simulink library "asbhl20act"  (R2016b)
settings: Solver=ode45  StartTime=0.0  StopTime=10.0  RelTol=1e-3
undefined symbols (not defined in the file): max_lim, min_lim
libraries: aerolibactuator x13, simulink x12
Description:
  | HL-20 control surface actuators component module
  | 
  | Copyright 1990-2007 The MathWorks Inc.
settings Model: Creator=The MathWorks, Inc.  LastModifiedBy=The MathWorks, Inc.
settings DataIOCC: LimitDataPoints=on  SaveFormat=Array  SignalLoggingSaveFormat=ModelDataLogs
settings OptimizationCC: BlockReduction=off  BooleanDataType=off  ExpressionDepthLimit=2147483647  LifeSpan=inf
settings DebuggingCC: SaveWithParameterizedLinksMsg=none  UnderspecifiedInitializationDetection=Classic  MergeDetectMultiDrivingBlocksExec=none  SignalResolutionControl=TryResolveAllWithWarning  MultiTaskCondExecSysMsg=none  FcnCallInpInsideContextMsg=warning  StateNameClashWarn=warning  StrictBusMsg=None  SFUnexpectedBacktrackingDiag=warning  SFNoUnconditionalDefaultTransitionDiag=warning  SFExecutionAtInitializationDiag=none
settings HardwareCC: ProdBitPerPointer=32  ProdBitPerSizeT=32  ProdBitPerPtrDiffT=32  ProdLargestAtomicFloat=None  ProdIntDivRoundTo=Undefined  ProdEndianess=Unspecified  ProdWordSize=32  ProdHWDeviceType=32-bit Generic  TargetUnknown=on
settings ModelReferenceCC: PropagateSignalLabelsOutOfModel=off
settings GRTTargetCC: TargetLangStandard=C89/C90 (ANSI)  GeneratePreprocessorConditionals=Disable all  CombineOutputUpdateFcns=off  GRTInterface=on
settings ConfigComp: CovMetricSettings=dw  CovHtmlReporting=on  CovSaveCumulativeToWorkspaceVar=on  CovSaveSingleToWorkspaceVar=on  CovExternalEMLEnable=off

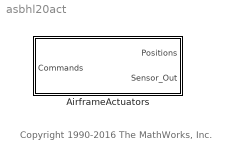
== system asbhl20act ==
  note: Copyright 1990-2016 The MathWorks, Inc.
  AirframeActuators : Subsystem

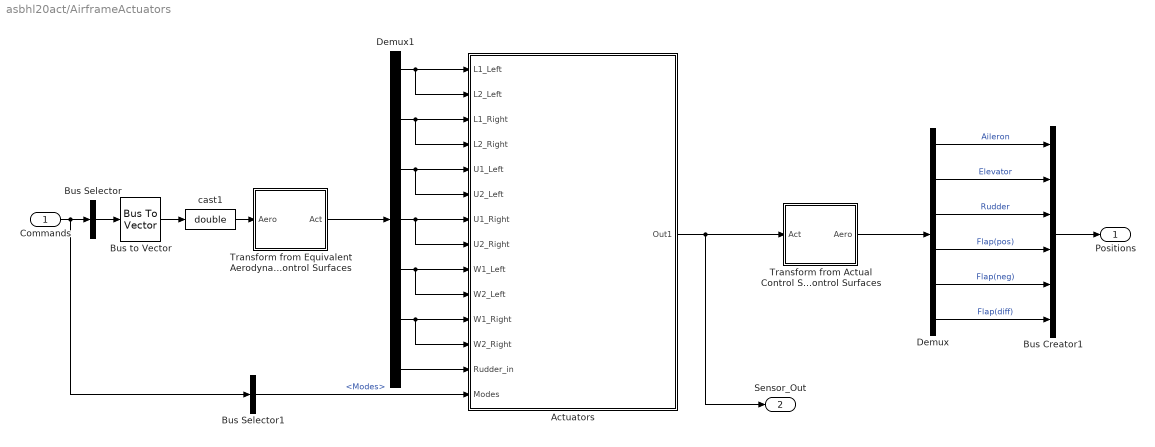
== system asbhl20act/AirframeActuators ==
  Commands : Inport
  Actuators : Subsystem
  Bus Creator1 : BusCreator  Inputs=6
  Bus Selector : BusSelector  OutputSignals=Aileron,Elevator,Rudder,Pos_flap,Neg_flap,Diff_flap  OutputAsBus=on
  Bus Selector1 : BusSelector  OutputSignals=Modes
  Bus to Vector : BusToVector
  Demux : Demux  Outputs=6
  Demux1 : Demux  Outputs=7
  Transform from Actual Control Surfaces to Equivalent Aerodynamic Control Surfaces : Subsystem
  Transform from Equivalent Aerodynamic Control Surfaces to Actual Control Surfaces : Subsystem
  cast1 : DataTypeConversion  OutDataTypeStr=double  SaturateOnIntegerOverflow=on  RndMeth=Zero
  Positions : Outport
  Sensor_Out : Outport  Port=2
  wires:
  Bus Selector1/1 -> Actuators/14(Modes)  "<Modes>"
  Bus Selector/1 -> Bus to Vector/1
  cast1/1 -> Transform from Equivalent Aerodynamic Control Surfaces to Actual Control Surfaces/1(Aero)
  Demux/1 -> Bus Creator1/1  "Aileron"
  Demux/2 -> Bus Creator1/2  "Elevator"
  Demux/3 -> Bus Creator1/3  "Rudder"
  Demux/4 -> Bus Creator1/4  "Flap(pos)"
  Demux/5 -> Bus Creator1/5  "Flap(neg)"
  Demux/6 -> Bus Creator1/6  "Flap(diff)"
  Bus Creator1/1 -> Positions/1
  Transform from Actual Control Surfaces to Equivalent Aerodynamic Control Surfaces/1(Aero) -> Demux/1
  Commands/1 -> Bus Selector1/1, Bus Selector/1
  Transform from Equivalent Aerodynamic Control Surfaces to Actual Control Surfaces/1(Act) -> Demux1/1
  Demux1/1 -> Actuators/1(L1_Left), Actuators/2(L2_Left)
  Demux1/2 -> Actuators/3(L1_Right), Actuators/4(L2_Right)
  Demux1/3 -> Actuators/5(U1_Left), Actuators/6(U2_Left)
  Demux1/4 -> Actuators/7(U1_Right), Actuators/8(U2_Right)
  Demux1/5 -> Actuators/9(W1_Left), Actuators/10(W2_Left)
  Demux1/6 -> Actuators/11(W1_Right), Actuators/12(W2_Right)
  Demux1/7 -> Actuators/13(Rudder_in)
  Actuators/1(Out1) -> Transform from Actual Control Surfaces to Equivalent Aerodynamic Control Surfaces/1(Act), Sensor_Out/1
  Bus to Vector/1 -> cast1/1

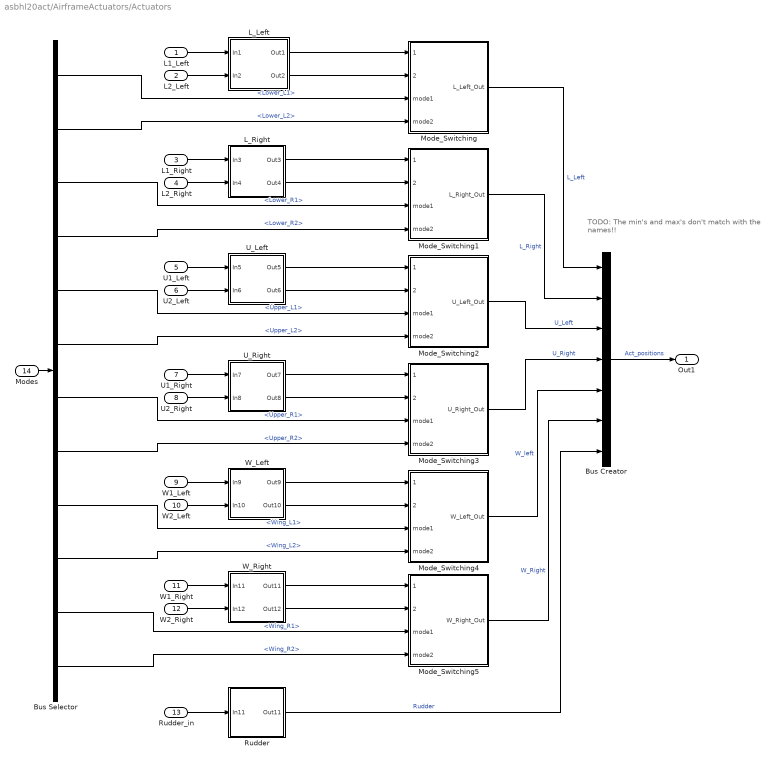
== system asbhl20act/AirframeActuators/Actuators ==
  note: TODO:
      | The min's and max's don't match with the names!!
  L1_Left : Inport
  L2_Left : Inport  Port=2
  L1_Right : Inport  Port=3
  L2_Right : Inport  Port=4
  U1_Left : Inport  Port=5
  U2_Left : Inport  Port=6
  U1_Right : Inport  Port=7
  U2_Right : Inport  Port=8
  W1_Left : Inport  Port=9
  W2_Left : Inport  Port=10
  W1_Right : Inport  Port=11
  W2_Right : Inport  Port=12
  Rudder_in : Inport  Port=13
  Modes : Inport  Port=14
  Bus Creator : BusCreator  Inputs=7
  Bus Selector : BusSelector  OutputSignals=Lower_L1,Lower_L2,Lower_R1,Lower_R2,Upper_L1,Upper_L2,Upper_R1,Upper_R2,Wing_L1,Wing_L2,Wing_R1,Wing_R2
  L_Left : Subsystem
  L_Right : Subsystem
  Mode_Switching : Subsystem
  Mode_Switching1 : Subsystem
  Mode_Switching2 : Subsystem
  Mode_Switching3 : Subsystem
  Mode_Switching4 : Subsystem
  Mode_Switching5 : Subsystem
  Rudder : Subsystem
  U_Left : Subsystem
  U_Right : Subsystem
  W_Left : Subsystem
  W_Right : Subsystem
  Out1 : Outport
  wires:
  L1_Left/1 -> L_Left/1(In1)
  L2_Left/1 -> L_Left/2(In2)
  L1_Right/1 -> L_Right/1(In3)
  L2_Right/1 -> L_Right/2(In4)
  U1_Left/1 -> U_Left/1(In5)
  U2_Left/1 -> U_Left/2(In6)
  U1_Right/1 -> U_Right/1(In7)
  U2_Right/1 -> U_Right/2(In8)
  W1_Left/1 -> W_Left/1(In9)
  W2_Left/1 -> W_Left/2(In10)
  W1_Right/1 -> W_Right/1(In11)
  W2_Right/1 -> W_Right/2(In12)
  Rudder_in/1 -> Rudder/1(In11)
  Modes/1 -> Bus Selector/1
  Bus Selector/1 -> Mode_Switching/3(mode1)  "<Lower_L1>"
  Bus Selector/2 -> Mode_Switching/4(mode2)  "<Lower_L2>"
  L_Left/1(Out1) -> Mode_Switching/1(1)
  L_Left/2(Out2) -> Mode_Switching/2(2)
  L_Right/1(Out3) -> Mode_Switching1/1(1)
  L_Right/2(Out4) -> Mode_Switching1/2(2)
  U_Left/1(Out5) -> Mode_Switching2/1(1)
  U_Left/2(Out6) -> Mode_Switching2/2(2)
  U_Right/1(Out7) -> Mode_Switching3/1(1)
  U_Right/2(Out8) -> Mode_Switching3/2(2)
  W_Left/1(Out9) -> Mode_Switching4/1(1)
  W_Left/2(Out10) -> Mode_Switching4/2(2)
  W_Right/1(Out11) -> Mode_Switching5/1(1)
  W_Right/2(Out12) -> Mode_Switching5/2(2)
  Bus Selector/3 -> Mode_Switching1/3(mode1)  "<Lower_R1>"
  Bus Selector/4 -> Mode_Switching1/4(mode2)  "<Lower_R2>"
  Bus Selector/5 -> Mode_Switching2/3(mode1)  "<Upper_L1>"
  Bus Selector/6 -> Mode_Switching2/4(mode2)  "<Upper_L2>"
  Bus Selector/7 -> Mode_Switching3/3(mode1)  "<Upper_R1>"
  Bus Selector/8 -> Mode_Switching3/4(mode2)  "<Upper_R2>"
  Bus Selector/9 -> Mode_Switching4/3(mode1)  "<Wing_L1>"
  Bus Selector/10 -> Mode_Switching4/4(mode2)  "<Wing_L2>"
  Bus Selector/11 -> Mode_Switching5/3(mode1)  "<Wing_R1>"
  Bus Selector/12 -> Mode_Switching5/4(mode2)  "<Wing_R2>"
  Mode_Switching/1(L_Left_Out) -> Bus Creator/1  "L_Left"
  Mode_Switching1/1(L_Right_Out) -> Bus Creator/2  "L_Right"
  Mode_Switching2/1(U_Left_Out) -> Bus Creator/3  "U_Left"
  Mode_Switching3/1(U_Right_Out) -> Bus Creator/4  "U_Right"
  Mode_Switching4/1(W_Left_Out) -> Bus Creator/5  "W_left"
  Mode_Switching5/1(W_Right_Out) -> Bus Creator/6  "W_Right"
  Rudder/1(Out11) -> Bus Creator/7  "Rudder"
  Bus Creator/1 -> Out1/1  "Act_positions"

== system asbhl20act/AirframeActuators/Transform from Actual Control Surfaces to Equivalent Aerodynamic Control Surfaces ==
  Act : Inport
  Bus to Vector : BusToVector
  Constant : Constant  Value="[0.5 -0.5 0 0 0 0 0; 0.5 0.5 0 0 0 0 0; 0 0 0 0 0 0 1;0 0 0.5 0.5 0 0 0; 0 0 0 0  0.5  0.5 0;0 0 0.5 -0.5 0.5 -0.5 0]"
  Product : Product  Multiplication=Matrix(*)  RndMeth=Zero
  Aero : Outport
  wires:
  Act/1 -> Bus to Vector/1
  Product/1 -> Aero/1
  Constant/1 -> Product/1
  Bus to Vector/1 -> Product/2

== system asbhl20act/AirframeActuators/Transform from Equivalent Aerodynamic Control Surfaces to Actual Control Surfaces ==
  Aero : Inport
  Constant : Constant  Value="[1 1  0 0 0 0; -1 1 0 0 0 0; 0 0 0 1 0 0.5; 0 0 0 1 0 -0.5;0 0 0 0 1 0.5; 0 0 0 0 1 -0.5;0 0 1 0 0 0]"
  Product : Product  Multiplication=Matrix(*)  RndMeth=Zero
  Act : Outport
  wires:
  Constant/1 -> Product/1
  Product/1 -> Act/1
  Aero/1 -> Product/2

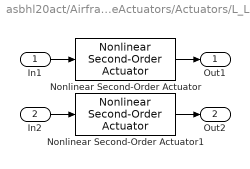
== system asbhl20act/AirframeActuators/Actuators/L_Left ==
  In1 : Inport
  In2 : Inport  Port=2
  Nonlinear Second-Order Actuator : aerolibactuator/Nonlinear Second-Order Actuator  wn_fin=wn_act  z_fin=z_act  fin_max=max_lim(1)  fin_min=min_lim(1)  fin_maxrate=Inf  fin_act_0=0  fin_act_vel=0
  Nonlinear Second-Order Actuator1 : aerolibactuator/Nonlinear Second-Order Actuator  wn_fin=wn_act  z_fin=z_act  fin_max=max_lim(1)  fin_min=min_lim(1)  fin_maxrate=Inf  fin_act_0=0  fin_act_vel=0
  Out1 : Outport
  Out2 : Outport  Port=2
  wires:
  In1/1 -> Nonlinear Second-Order Actuator/1
  Nonlinear Second-Order Actuator/1 -> Out1/1
  In2/1 -> Nonlinear Second-Order Actuator1/1
  Nonlinear Second-Order Actuator1/1 -> Out2/1

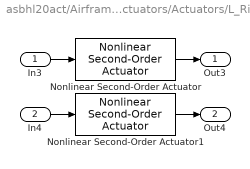
== system asbhl20act/AirframeActuators/Actuators/L_Right ==
  In3 : Inport
  In4 : Inport  Port=2
  Nonlinear Second-Order Actuator : aerolibactuator/Nonlinear Second-Order Actuator  wn_fin=wn_act  z_fin=z_act  fin_max=max_lim(2)  fin_min=min_lim(2)  fin_maxrate=Inf  fin_act_0=0  fin_act_vel=0
  Nonlinear Second-Order Actuator1 : aerolibactuator/Nonlinear Second-Order Actuator  wn_fin=wn_act  z_fin=z_act  fin_max=max_lim(2)  fin_min=min_lim(2)  fin_maxrate=Inf  fin_act_0=0  fin_act_vel=0
  Out3 : Outport
  Out4 : Outport  Port=2
  wires:
  In3/1 -> Nonlinear Second-Order Actuator/1
  Nonlinear Second-Order Actuator/1 -> Out3/1
  In4/1 -> Nonlinear Second-Order Actuator1/1
  Nonlinear Second-Order Actuator1/1 -> Out4/1

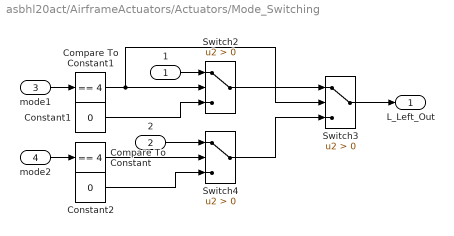
== system asbhl20act/AirframeActuators/Actuators/Mode_Switching ==
  1 : Inport
  2 : Inport  Port=2
  mode1 : Inport  Port=3
  mode2 : Inport  Port=4
  Compare To Constant : simulink/Logic and Bit Operations/Compare To Constant  relop===  const=4  OutDataTypeStr=uint8
  Compare To Constant1 : simulink/Logic and Bit Operations/Compare To Constant  relop===  const=4  OutDataTypeStr=uint8
  Constant1 : Constant  Value=0
  Constant2 : Constant  Value=0
  Switch2 : Switch  Criteria=u2 > Threshold
  Switch3 : Switch  Criteria=u2 > Threshold
  Switch4 : Switch  Criteria=u2 > Threshold
  L_Left_Out : Outport
  wires:
  Switch3/1 -> L_Left_Out/1
  Compare To Constant1/1 -> Switch2/2, Switch3/2
  Constant1/1 -> Switch2/3
  Compare To Constant/1 -> Switch4/2
  Constant2/1 -> Switch4/3
  1/1 -> Switch2/1
  mode1/1 -> Compare To Constant1/1
  2/1 -> Switch4/1
  mode2/1 -> Compare To Constant/1
  Switch2/1 -> Switch3/1
  Switch4/1 -> Switch3/3

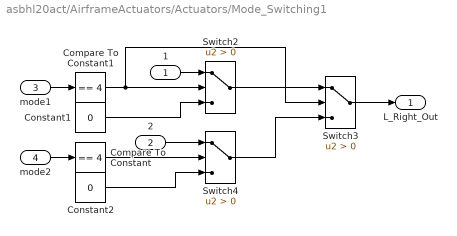
== system asbhl20act/AirframeActuators/Actuators/Mode_Switching1 ==
  1 : Inport
  2 : Inport  Port=2
  mode1 : Inport  Port=3
  mode2 : Inport  Port=4
  Compare To Constant : simulink/Logic and Bit Operations/Compare To Constant  relop===  const=4  OutDataTypeStr=uint8
  Compare To Constant1 : simulink/Logic and Bit Operations/Compare To Constant  relop===  const=4  OutDataTypeStr=uint8
  Constant1 : Constant  Value=0
  Constant2 : Constant  Value=0
  Switch2 : Switch  Criteria=u2 > Threshold
  Switch3 : Switch  Criteria=u2 > Threshold
  Switch4 : Switch  Criteria=u2 > Threshold
  L_Right_Out : Outport
  wires:
  Switch4/1 -> Switch3/3
  Switch2/1 -> Switch3/1
  mode2/1 -> Compare To Constant/1
  2/1 -> Switch4/1
  mode1/1 -> Compare To Constant1/1
  1/1 -> Switch2/1
  Constant2/1 -> Switch4/3
  Compare To Constant/1 -> Switch4/2
  Constant1/1 -> Switch2/3
  Compare To Constant1/1 -> Switch3/2, Switch2/2
  Switch3/1 -> L_Right_Out/1

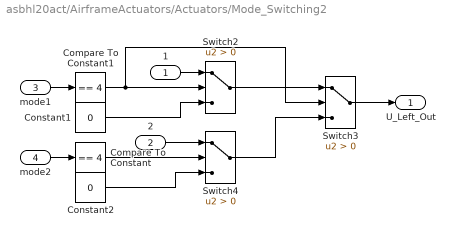
== system asbhl20act/AirframeActuators/Actuators/Mode_Switching2 ==
  1 : Inport
  2 : Inport  Port=2
  mode1 : Inport  Port=3
  mode2 : Inport  Port=4
  Compare To Constant : simulink/Logic and Bit Operations/Compare To Constant  relop===  const=4  OutDataTypeStr=uint8
  Compare To Constant1 : simulink/Logic and Bit Operations/Compare To Constant  relop===  const=4  OutDataTypeStr=uint8
  Constant1 : Constant  Value=0
  Constant2 : Constant  Value=0
  Switch2 : Switch  Criteria=u2 > Threshold
  Switch3 : Switch  Criteria=u2 > Threshold
  Switch4 : Switch  Criteria=u2 > Threshold
  U_Left_Out : Outport
  wires:
  Switch3/1 -> U_Left_Out/1
  Compare To Constant1/1 -> Switch2/2, Switch3/2
  Constant1/1 -> Switch2/3
  Compare To Constant/1 -> Switch4/2
  Constant2/1 -> Switch4/3
  1/1 -> Switch2/1
  mode1/1 -> Compare To Constant1/1
  2/1 -> Switch4/1
  mode2/1 -> Compare To Constant/1
  Switch2/1 -> Switch3/1
  Switch4/1 -> Switch3/3

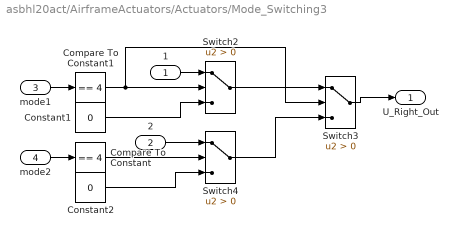
== system asbhl20act/AirframeActuators/Actuators/Mode_Switching3 ==
  1 : Inport
  2 : Inport  Port=2
  mode1 : Inport  Port=3
  mode2 : Inport  Port=4
  Compare To Constant : simulink/Logic and Bit Operations/Compare To Constant  relop===  const=4  OutDataTypeStr=uint8
  Compare To Constant1 : simulink/Logic and Bit Operations/Compare To Constant  relop===  const=4  OutDataTypeStr=uint8
  Constant1 : Constant  Value=0
  Constant2 : Constant  Value=0
  Switch2 : Switch  Criteria=u2 > Threshold
  Switch3 : Switch  Criteria=u2 > Threshold
  Switch4 : Switch  Criteria=u2 > Threshold
  U_Right_Out : Outport
  wires:
  Switch3/1 -> U_Right_Out/1
  Compare To Constant1/1 -> Switch2/2, Switch3/2
  Constant1/1 -> Switch2/3
  Compare To Constant/1 -> Switch4/2
  Constant2/1 -> Switch4/3
  1/1 -> Switch2/1
  mode1/1 -> Compare To Constant1/1
  2/1 -> Switch4/1
  mode2/1 -> Compare To Constant/1
  Switch2/1 -> Switch3/1
  Switch4/1 -> Switch3/3

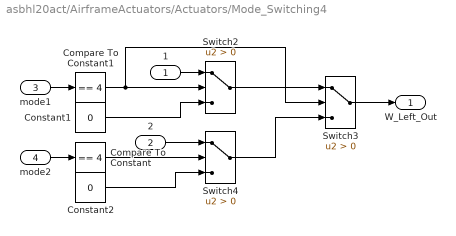
== system asbhl20act/AirframeActuators/Actuators/Mode_Switching4 ==
  1 : Inport
  2 : Inport  Port=2
  mode1 : Inport  Port=3
  mode2 : Inport  Port=4
  Compare To Constant : simulink/Logic and Bit Operations/Compare To Constant  relop===  const=4  OutDataTypeStr=uint8
  Compare To Constant1 : simulink/Logic and Bit Operations/Compare To Constant  relop===  const=4  OutDataTypeStr=uint8
  Constant1 : Constant  Value=0
  Constant2 : Constant  Value=0
  Switch2 : Switch  Criteria=u2 > Threshold
  Switch3 : Switch  Criteria=u2 > Threshold
  Switch4 : Switch  Criteria=u2 > Threshold
  W_Left_Out : Outport
  wires:
  Switch4/1 -> Switch3/3
  Switch2/1 -> Switch3/1
  mode2/1 -> Compare To Constant/1
  2/1 -> Switch4/1
  mode1/1 -> Compare To Constant1/1
  1/1 -> Switch2/1
  Constant2/1 -> Switch4/3
  Compare To Constant/1 -> Switch4/2
  Constant1/1 -> Switch2/3
  Compare To Constant1/1 -> Switch3/2, Switch2/2
  Switch3/1 -> W_Left_Out/1

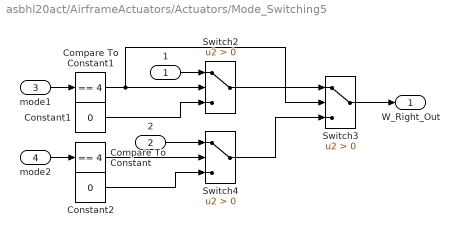
== system asbhl20act/AirframeActuators/Actuators/Mode_Switching5 ==
  1 : Inport
  2 : Inport  Port=2
  mode1 : Inport  Port=3
  mode2 : Inport  Port=4
  Compare To Constant : simulink/Logic and Bit Operations/Compare To Constant  relop===  const=4  OutDataTypeStr=uint8
  Compare To Constant1 : simulink/Logic and Bit Operations/Compare To Constant  relop===  const=4  OutDataTypeStr=uint8
  Constant1 : Constant  Value=0
  Constant2 : Constant  Value=0
  Switch2 : Switch  Criteria=u2 > Threshold
  Switch3 : Switch  Criteria=u2 > Threshold
  Switch4 : Switch  Criteria=u2 > Threshold
  W_Right_Out : Outport
  wires:
  Switch3/1 -> W_Right_Out/1
  Compare To Constant1/1 -> Switch2/2, Switch3/2
  Constant1/1 -> Switch2/3
  Compare To Constant/1 -> Switch4/2
  Constant2/1 -> Switch4/3
  1/1 -> Switch2/1
  mode1/1 -> Compare To Constant1/1
  2/1 -> Switch4/1
  mode2/1 -> Compare To Constant/1
  Switch2/1 -> Switch3/1
  Switch4/1 -> Switch3/3

== system asbhl20act/AirframeActuators/Actuators/Rudder ==
  In11 : Inport
  Nonlinear Second-Order Actuator1 : aerolibactuator/Nonlinear Second-Order Actuator  wn_fin=wn_act  z_fin=z_act  fin_max=max_lim(7)  fin_min=min_lim(7)  fin_maxrate=Inf  fin_act_0=0  fin_act_vel=0
  Out11 : Outport
  wires:
  Nonlinear Second-Order Actuator1/1 -> Out11/1
  In11/1 -> Nonlinear Second-Order Actuator1/1

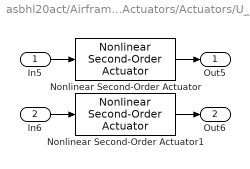
== system asbhl20act/AirframeActuators/Actuators/U_Left ==
  In5 : Inport
  In6 : Inport  Port=2
  Nonlinear Second-Order Actuator : aerolibactuator/Nonlinear Second-Order Actuator  wn_fin=wn_act  z_fin=z_act  fin_max=max_lim(3)  fin_min=min_lim(3)  fin_maxrate=Inf  fin_act_0=0  fin_act_vel=0
  Nonlinear Second-Order Actuator1 : aerolibactuator/Nonlinear Second-Order Actuator  wn_fin=wn_act  z_fin=z_act  fin_max=max_lim(3)  fin_min=min_lim(3)  fin_maxrate=Inf  fin_act_0=0  fin_act_vel=0
  Out5 : Outport
  Out6 : Outport  Port=2
  wires:
  In5/1 -> Nonlinear Second-Order Actuator/1
  Nonlinear Second-Order Actuator/1 -> Out5/1
  In6/1 -> Nonlinear Second-Order Actuator1/1
  Nonlinear Second-Order Actuator1/1 -> Out6/1

== system asbhl20act/AirframeActuators/Actuators/U_Right ==
  In7 : Inport
  In8 : Inport  Port=2
  Nonlinear Second-Order Actuator : aerolibactuator/Nonlinear Second-Order Actuator  wn_fin=wn_act  z_fin=z_act  fin_max=max_lim(4)  fin_min=min_lim(4)  fin_maxrate=Inf  fin_act_0=0  fin_act_vel=0
  Nonlinear Second-Order Actuator1 : aerolibactuator/Nonlinear Second-Order Actuator  wn_fin=wn_act  z_fin=z_act  fin_max=max_lim(4)  fin_min=min_lim(4)  fin_maxrate=Inf  fin_act_0=0  fin_act_vel=0
  Out7 : Outport
  Out8 : Outport  Port=2
  wires:
  In7/1 -> Nonlinear Second-Order Actuator/1
  Nonlinear Second-Order Actuator/1 -> Out7/1
  In8/1 -> Nonlinear Second-Order Actuator1/1
  Nonlinear Second-Order Actuator1/1 -> Out8/1

== system asbhl20act/AirframeActuators/Actuators/W_Left ==
  In9 : Inport
  In10 : Inport  Port=2
  Nonlinear Second-Order Actuator : aerolibactuator/Nonlinear Second-Order Actuator  wn_fin=wn_act  z_fin=z_act  fin_max=max_lim(5)  fin_min=min_lim(5)  fin_maxrate=Inf  fin_act_0=0  fin_act_vel=0
  Nonlinear Second-Order Actuator1 : aerolibactuator/Nonlinear Second-Order Actuator  wn_fin=wn_act  z_fin=z_act  fin_max=max_lim(5)  fin_min=min_lim(5)  fin_maxrate=Inf  fin_act_0=0  fin_act_vel=0
  Out9 : Outport
  Out10 : Outport  Port=2
  wires:
  In9/1 -> Nonlinear Second-Order Actuator/1
  Nonlinear Second-Order Actuator/1 -> Out9/1
  In10/1 -> Nonlinear Second-Order Actuator1/1
  Nonlinear Second-Order Actuator1/1 -> Out10/1

== system asbhl20act/AirframeActuators/Actuators/W_Right ==
  In11 : Inport
  In12 : Inport  Port=2
  Nonlinear Second-Order Actuator : aerolibactuator/Nonlinear Second-Order Actuator  wn_fin=wn_act  z_fin=z_act  fin_max=max_lim(6)  fin_min=min_lim(6)  fin_maxrate=Inf  fin_act_0=0  fin_act_vel=0
  Nonlinear Second-Order Actuator1 : aerolibactuator/Nonlinear Second-Order Actuator  wn_fin=wn_act  z_fin=z_act  fin_max=max_lim(6)  fin_min=min_lim(6)  fin_maxrate=Inf  fin_act_0=0  fin_act_vel=0
  Out11 : Outport
  Out12 : Outport  Port=2
  wires:
  In11/1 -> Nonlinear Second-Order Actuator/1
  Nonlinear Second-Order Actuator/1 -> Out11/1
  In12/1 -> Nonlinear Second-Order Actuator1/1
  Nonlinear Second-Order Actuator1/1 -> Out12/1
